simulink model "maglev_Controller_Linear_System"  (R2021b)
settings: Solver=ode45  StartTime=0.0  StopTime=Tsim  RelTol=1e-3  EnableMultiTasking=on
undefined symbols (not defined in the file): Ae, Be, Ce, De, K, kalmf, Lc
settings Model: Creator=rbabuska  LastModifiedBy=tlijding
settings SolverCC: AlgebraicLoopSolver=TrustRegion
settings DataIOCC: LimitDataPoints=on  SaveFormat=Array  ReturnWorkspaceOutputs=off
settings OptimizationCC: ExpressionDepthLimit=2147483647  InitFltsAndDblsToZero=on  LifeSpan=inf
settings DebuggingCC: SaveWithParameterizedLinksMsg=none  SignalResolutionControl=TryResolveAllWithWarning  SolverPrmCheckMsg=warning  MultiTaskCondExecSysMsg=none  AllowSymbolicDim=off  StateNameClashWarn=warning  StrictBusMsg=ErrorOnBusTreatedAsVector  SFUnexpectedBacktrackingDiag=warning  SFNoUnconditionalDefaultTransitionDiag=warning  SFExecutionAtInitializationDiag=none  SFMachineParentedDataDiag=warning  ArithmeticOperatorsInVariantConditions=warning
settings HardwareCC: ProdBitPerPointer=32  ProdBitPerSizeT=32  ProdBitPerPtrDiffT=32  ProdLargestAtomicFloat=None  ProdIntDivRoundTo=Undefined  ProdEndianess=Unspecified  ProdWordSize=32  ProdHWDeviceType=32-bit Generic
settings ModelReferenceCC: PropagateSignalLabelsOutOfModel=off
settings SFSimCC: SimUseLocalCustomCode=off  CustomCodeUndefinedFunction=UseInterfaceOnly
settings RTWCC: RTWUseLocalCustomCode=off
settings CodeAppCC: StateflowObjectComments=on
settings GRTTargetCC: TargetFcnLib=ansi_tfl_tmw.mat  TargetLangStandard=C89/C90 (ANSI)  CombineOutputUpdateFcns=off  GRTInterface=on
settings ConfigComp: CovMetricSettings=dw  CovSaveCumulativeToWorkspaceVar=on  CovSaveSingleToWorkspaceVar=on  CovExternalEMLEnable=off  CovSFcnEnable=off

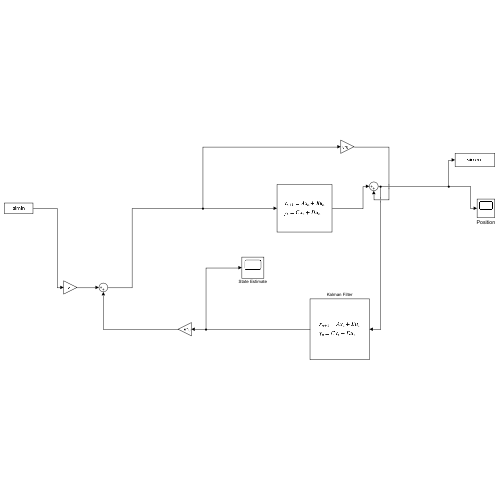
[thumbnail: Simulink's stored preview of the top-level diagram]
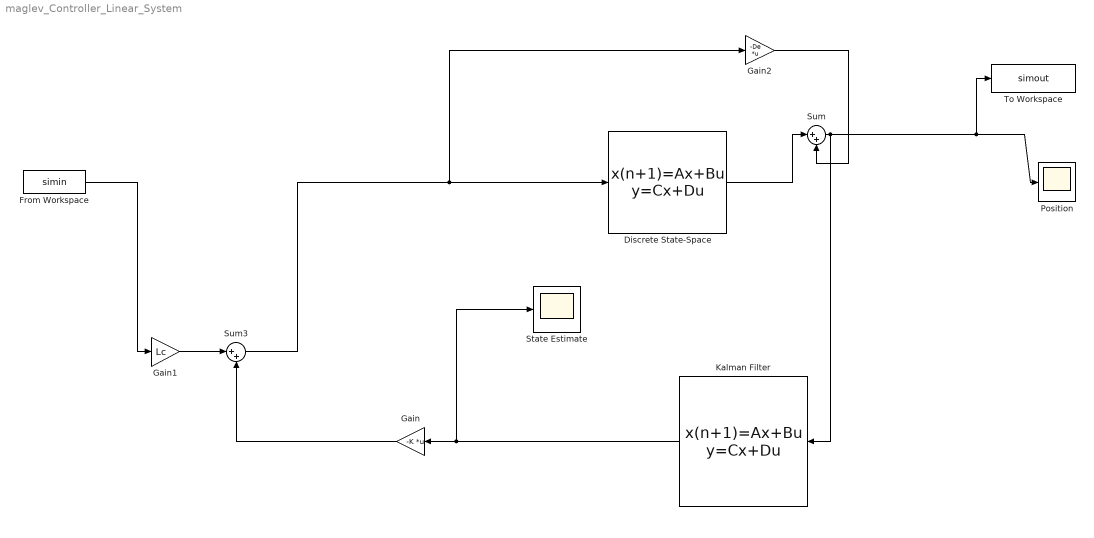
== system maglev_Controller_Linear_System ==
  Discrete State-Space : DiscreteStateSpace  A=Ae  B=Be  C=Ce  D=De  InitialCondition=[0.1 0.1 0.1]  SampleTime=-1
  From Workspace : FromWorkspace  VariableName=simin
  Gain : Gain  Gain=-K  Multiplication=Matrix(K*u)
  Gain1 : Gain  Gain=Lc
  Gain2 : Gain  Gain=-De  Multiplication=Matrix(K*u)
  Kalman Filter : DiscreteStateSpace  A=kalmf.A  B=kalmf.B  C=kalmf.C  D=kalmf.D  SampleTime=-1  StateName=Kalman Filter
  Position : Scope
  State Estimate : Scope
  Sum : Sum  Inputs=|++
  Sum3 : Sum  Inputs=|++
  To Workspace : ToWorkspace  VariableName=simout  SaveFormat=Timeseries  SampleTime=-1
  wires:
  Discrete State-Space/1 -> Sum/1
  Sum3/1 -> Discrete State-Space/1, Gain2/1
  From Workspace/1 -> Gain1/1
  Kalman Filter/1 -> Gain/1, State Estimate/1
  Gain/1 -> Sum3/2
  Gain1/1 -> Sum3/1
  Gain2/1 -> Sum/2
  Sum/1 -> Kalman Filter/1, To Workspace/1, Position/1
